simulink model "SimulacionSisElectrico"  (R2024a)
settings: Solver=VariableStepAuto  StartTime=0.0  StopTime=100  RelTol=1e-3
libraries: simulink x1
settings Model: Creator=sebas  LastModifiedBy=andre
settings RTWCC: GPUComputeCapability=3.5

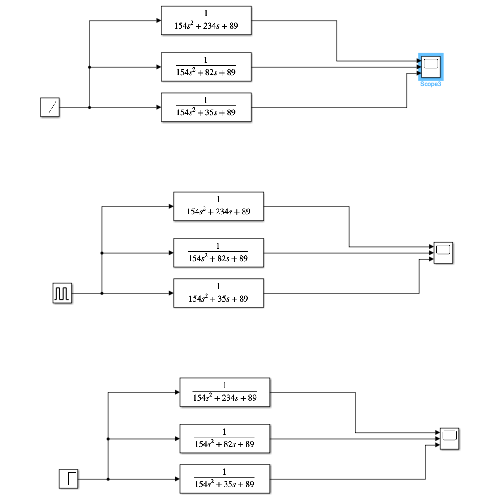
[thumbnail: Simulink's stored preview of the top-level diagram]
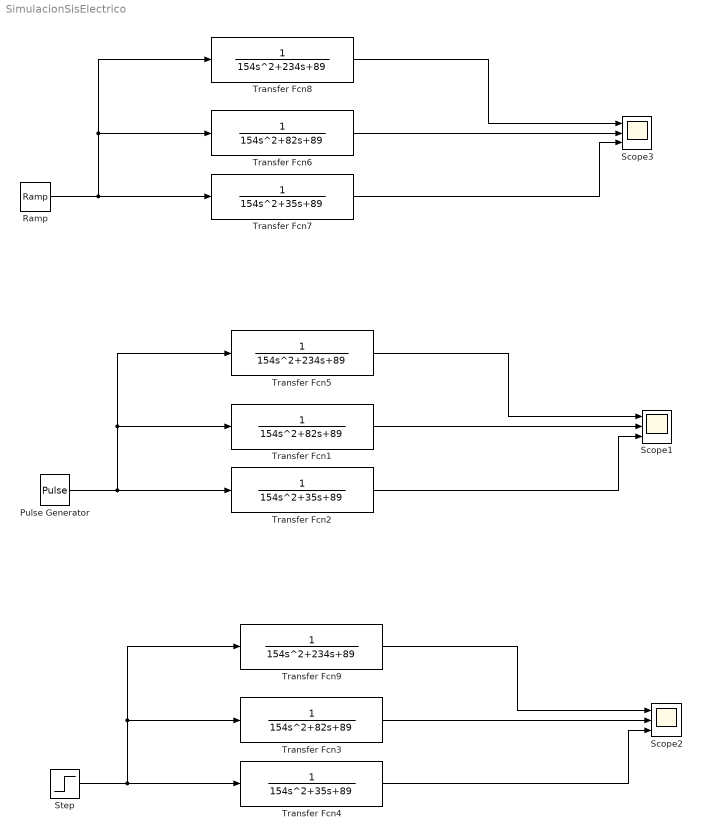
== system SimulacionSisElectrico ==
  Pulse Generator : DiscretePulseGenerator  PulseType=Time based  Period=10  PulseWidth=5
  Ramp : simulink/Sources/Ramp  slope=1  start=0  InitialOutput=0
  Scope1 : Scope  NumInputPorts=3
  Scope2 : Scope  NumInputPorts=3
  Scope3 : Scope  NumInputPorts=3
  Step : Step  Time=0  SampleTime=0
  Transfer Fcn1 : TransferFcn  Denominator="[154 82  89]"
  Transfer Fcn2 : TransferFcn  Denominator="[154 35  89]"
  Transfer Fcn3 : TransferFcn  Denominator="[154 82  89]"
  Transfer Fcn4 : TransferFcn  Denominator="[154 35  89]"
  Transfer Fcn5 : TransferFcn  Denominator="[154 234  89]"
  Transfer Fcn6 : TransferFcn  Denominator="[154 82  89]"
  Transfer Fcn7 : TransferFcn  Denominator="[154 35  89]"
  Transfer Fcn8 : TransferFcn  Denominator="[154 234  89]"
  Transfer Fcn9 : TransferFcn  Denominator="[154 234  89]"
  wires:
  Transfer Fcn4/1 -> Scope2/3
  Transfer Fcn9/1 -> Scope2/1
  Transfer Fcn3/1 -> Scope2/2
  Step/1 -> Transfer Fcn4/1, Transfer Fcn9/1, Transfer Fcn3/1
  Transfer Fcn2/1 -> Scope1/3
  Transfer Fcn5/1 -> Scope1/1
  Pulse Generator/1 -> Transfer Fcn2/1, Transfer Fcn5/1, Transfer Fcn1/1
  Transfer Fcn1/1 -> Scope1/2
  Transfer Fcn7/1 -> Scope3/3
  Transfer Fcn8/1 -> Scope3/1
  Ramp/1 -> Transfer Fcn7/1, Transfer Fcn8/1, Transfer Fcn6/1
  Transfer Fcn6/1 -> Scope3/2
